simulink model "maskExprHandling_example"  (R2018b)
settings: Solver=FixedStepDiscrete  StartTime=0.0  StopTime=10.0  FixedStep=ts  RelTol=1e-3
values from neighbouring files (symbols this model uses):
  ts = 0.0025    [init_maskExprHandling_example.m]
undefined symbols (not defined in the file or in its folder): param
libraries: maskExprHandling_example_lib x4
settings Model: DataTypeOverride=Single  DataTypeOverrideAppliesTo=Floating-point  TunableVars=param  TunableVarsStorageClass=Auto  Creator=jonas  LastModifiedBy=jonas
settings OptimizationCC: DefaultParameterBehavior=Inlined  UseFloatMulNetSlope=on  DefaultUnderspecifiedDataType=single  PassReuseOutputArgsAs=Individual arguments  ZeroExternalMemoryAtStartup=off  ZeroInternalMemoryAtStartup=off  OptimizeBlockOrder=speed  DifferentSizesBufferReuse=on
settings DebuggingCC: ParameterTunabilityLossMsg=error
settings HardwareCC: ProdBitPerPointer=32  ProdBitPerSizeT=32  ProdBitPerPtrDiffT=32  ProdLargestAtomicInteger=Long  ProdWordSize=32  ProdHWDeviceType=ARM Compatible->ARM 7
settings ModelReferenceCC: PropagateSignalLabelsOutOfModel=off
settings SFSimCC: MATLABDynamicMemAlloc=off
settings RTWCC: SystemTargetFile=ert.tlc  GenCodeOnly=on  TemplateMakefile=ert_default_tmf  GenerateReport=on  IncludeHyperlinkInReport=on  LaunchReport=on  TargetLang=C++  GenerateTraceInfo=on  GenerateTraceReport=on  GenerateTraceReportSl=on  GenerateTraceReportSf=on  GenerateTraceReportEml=on
settings CodeAppCC: ForceParamTrailComments=on  IgnoreCustomStorageClasses=off  OperatorAnnotations=on  SimulinkDataObjDesc=on  SFDataObjDesc=on  InsertBlockDesc=on
settings ERTTargetCC: TargetLangStandard=C++03 (ISO)  GenerateSampleERTMain=on  MultiInstanceERTCode=on  CodeInterfacePackaging=C++ class  SupportNonFinite=off  SupportComplex=off  SupportVariableSizeSignals=on  InlinedParameterPlacement=NonHierarchical  RootIOFormat=Structure reference  ERTCustomFileTemplate=example_file_process.tlc  ERTFilePackagingFormat=CompactWithDataFile  IndentSize=4

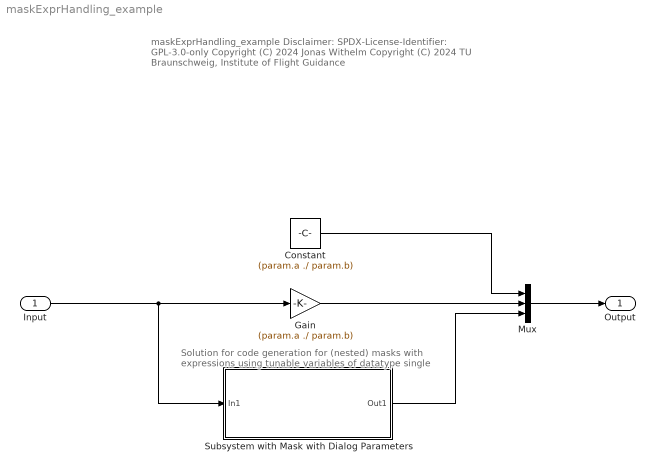
== system maskExprHandling_example ==
  note: Solution for code generation for (nested) masks with expressions using tunable variables of datatype single
  note: maskExprHandling_example
      |
      | Disclaimer:
      | SPDX-License-Identifier: GPL-3.0-only
      |
      | Copyright (C) 2024 Jonas Withelm
      | Copyright (C) 2024 TU Braunschweig, Institute of Flight Guidance
  Input : Inport
  Constant : Constant  Value=(param.a ./ param.b)  SampleTime=ts
  Gain : Gain  Gain=(param.a ./ param.b)
  Mux : Mux  Inputs=3
  Subsystem with Mask with Dialog Parameters : Subsystem  mask{par_a=param.a ./ param.b, mask_expr_handling_config=default}
      mask prompts: par_a "edit:"
      mask help: Just another mask
      mask init:
      | maskExprHandling(gcbh, mask_expr_handling_config);
      mask TypeOptions mask_expr_handling_config: default | passthrough (tunable)
      mask DialogControl CodeGenerationSettings Prompt: Code Generation Settings
      mask DialogControl maskExprHandlingText Prompt: Mask expression handling
      mask DialogControl maskExprHandlingReadme Prompt: README
      mask DialogControl maskExprHandlingReadme Tooltip: https://github.com/iff-gsc/m-Utils/tree/main/simulink/mask_expression_handling/README.md
      mask DialogControl maskExprHandlingReadme Callback: web('https://github.com/iff-gsc/m-Utils/tree/main/simulink/mask_expression_handling/README.md','-browser')
  Output : Outport
  wires:
  Input/1 -> Subsystem with Mask with Dialog Parameters/1(In1), Gain/1
  Gain/1 -> Mux/2
  Subsystem with Mask with Dialog Parameters/1(Out1) -> Mux/3
  Mux/1 -> Output/1
  Constant/1 -> Mux/1

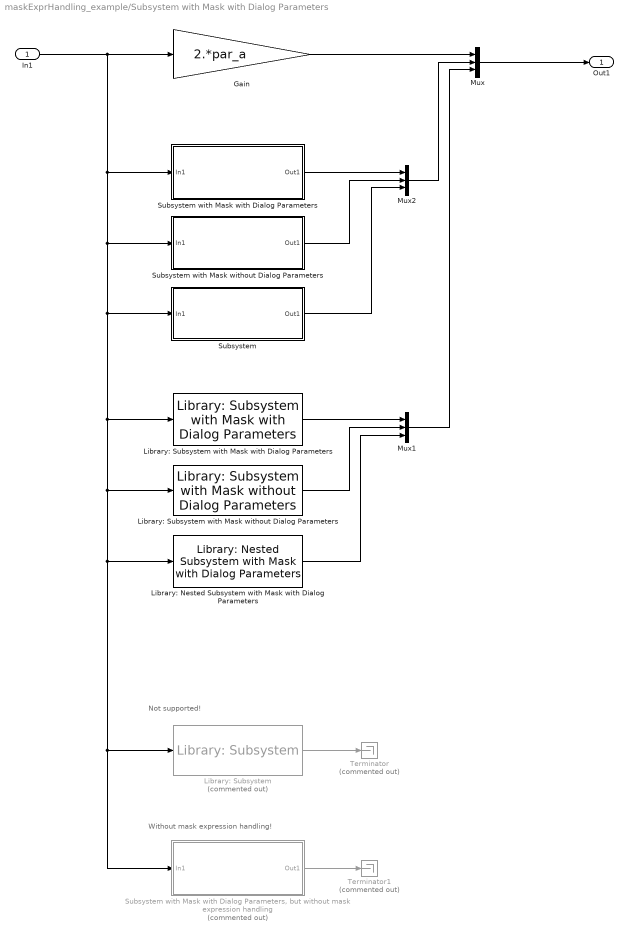
== system maskExprHandling_example/Subsystem with Mask with Dialog Parameters ==
  note: Not supported!
  note: Without mask expression handling!
  In1 : Inport
  Gain : Gain  Gain=2.*par_a
  Library: Nested Subsystem with Mask with Dialog Parameters : maskExprHandling_example_lib/Library: Nested Subsystem with Mask with Dialog Parameters  par_aa=2.*par_a  mask_expr_handling_config=default
  Library: Subsystem : maskExprHandling_example_lib/Library: Subsystem  Commented=on  SystemSampleTime=-1
  Library: Subsystem with Mask with Dialog Parameters : maskExprHandling_example_lib/Library: Subsystem with Mask with Dialog Parameters  par_aa=2.*par_a  mask_expr_handling_config=default
  Library: Subsystem with Mask without Dialog Parameters : maskExprHandling_example_lib/Library: Subsystem with Mask without Dialog Parameters  SystemSampleTime=-1
  Mux : Mux  Inputs=3
  Mux1 : Mux  Inputs=3
  Mux2 : Mux  Inputs=3
  Subsystem : Subsystem
  Subsystem with Mask with Dialog Parameters : Subsystem  mask{par_aa=2.*par_a, mask_expr_handling_config=default}
      mask prompts: par_aa "edit:"
      mask init:
      | maskExprHandling(gcbh, mask_expr_handling_config);
      mask TypeOptions mask_expr_handling_config: default | passthrough (tunable)
      mask DialogControl CodeGenerationSettings Prompt: Code Generation Settings
      mask DialogControl maskExprHandlingText Prompt: Mask expression handling
      mask DialogControl maskExprHandlingReadme Prompt: README
      mask DialogControl maskExprHandlingReadme Tooltip: https://github.com/iff-gsc/m-Utils/tree/main/simulink/mask_expression_handling/README.md
      mask DialogControl maskExprHandlingReadme Callback: web('https://github.com/iff-gsc/m-Utils/tree/main/simulink/mask_expression_handling/README.md','-browser')
  "Subsystem with Mask with Dialog Parameters, but without mask expression handling" : Subsystem  Commented=on  mask{par_aaplus=3.*par_a}
      mask prompts: par_aaplus "edit:"
  Subsystem with Mask without Dialog Parameters : Subsystem
  Terminator : Terminator  Commented=on
  Terminator1 : Terminator  Commented=on
  Out1 : Outport
  wires:
  Gain/1 -> Mux/1
  Mux/1 -> Out1/1
  Library: Subsystem with Mask with Dialog Parameters/1 -> Mux1/1
  Library: Subsystem with Mask without Dialog Parameters/1 -> Mux1/2
  Subsystem with Mask with Dialog Parameters/1(Out1) -> Mux2/1
  Subsystem with Mask without Dialog Parameters/1(Out1) -> Mux2/2
  Subsystem/1(Out1) -> Mux2/3
  Mux2/1 -> Mux/2
  Mux1/1 -> Mux/3
  In1/1 -> Library: Subsystem with Mask with Dialog Parameters/1, Library: Subsystem with Mask without Dialog Parameters/1, Library: Nested Subsystem with Mask with Dialog Parameters/1, Library: Subsystem/1, "Subsystem with Mask with Dialog Parameters, but without mask expression handling"/1(In1), Subsystem/1(In1), Subsystem with Mask without Dialog Parameters/1(In1), Subsystem with Mask with Dialog Parameters/1(In1), Gain/1
  Library: Nested Subsystem with Mask with Dialog Parameters/1 -> Mux1/3
  Library: Subsystem/1 -> Terminator/1
  "Subsystem with Mask with Dialog Parameters, but without mask expression handling"/1(Out1) -> Terminator1/1

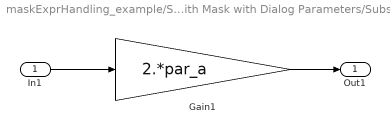
== system maskExprHandling_example/Subsystem with Mask with Dialog Parameters/Subsystem ==
  In1 : Inport
  Gain1 : Gain  Gain=2.*par_a
  Out1 : Outport
  wires:
  In1/1 -> Gain1/1
  Gain1/1 -> Out1/1

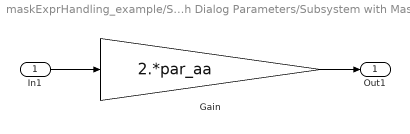
== system maskExprHandling_example/Subsystem with Mask with Dialog Parameters/Subsystem with Mask with Dialog Parameters ==
  In1 : Inport
  Gain : Gain  Gain=2.*par_aa
  Out1 : Outport
  wires:
  In1/1 -> Gain/1
  Gain/1 -> Out1/1

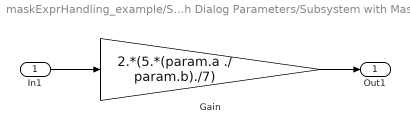
== system maskExprHandling_example/Subsystem with Mask with Dialog Parameters/Subsystem with Mask with Dialog Parameters, but without mask expression handling ==
  In1 : Inport
  Gain : Gain  Gain=2.*(5.*(param.a ./ param.b)./7)
  Out1 : Outport
  wires:
  In1/1 -> Gain/1
  Gain/1 -> Out1/1

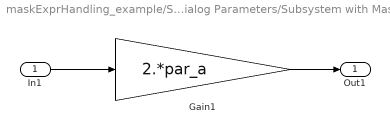
== system maskExprHandling_example/Subsystem with Mask with Dialog Parameters/Subsystem with Mask without Dialog Parameters ==
  In1 : Inport
  Gain1 : Gain  Gain=2.*par_a
  Out1 : Outport
  wires:
  Gain1/1 -> Out1/1
  In1/1 -> Gain1/1
